simulink model "CircuitoGlobal"  (R2018a)
settings: Solver=VariableStepAuto  StartTime=0.0  StopTime=10.0  RelTol=1e-3
libraries: powerlib x4, pePwmGenerator x1, simulink_extras x1
settings Model: Creator=MATHEUS  LastModifiedBy=MATHEUS

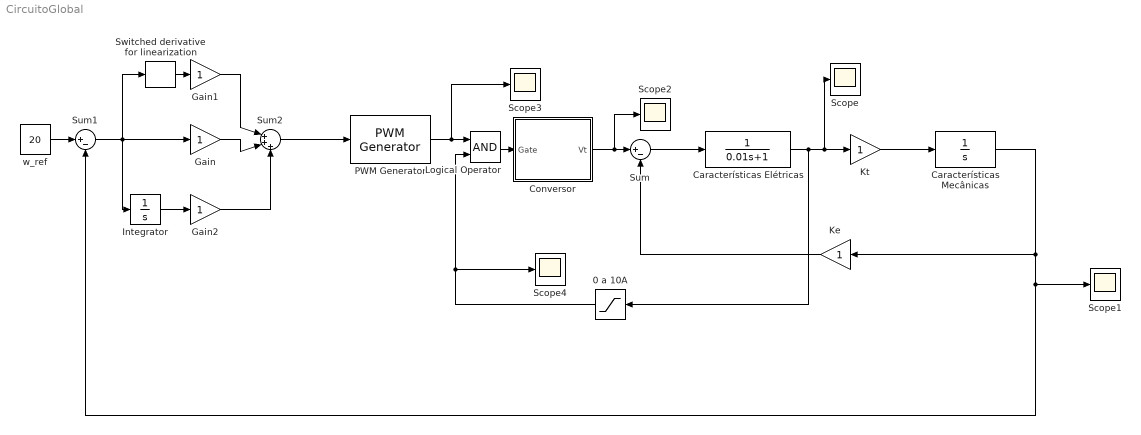
== system CircuitoGlobal ==
  0 a 10A : Saturate  UpperLimit=10  LowerLimit=0
  Características Elétricas : TransferFcn  Denominator=[0.01 1]
  "Características Mecânicas " : TransferFcn  Denominator=[1 0]
  Conversor : Subsystem
  Gain : Gain
  Gain1 : Gain
  Gain2 : Gain
  Integrator : Integrator
  Ke : Gain
  "Kt " : Gain
  Logical Operator : Logic  AllPortsSameDT=off  OutDataTypeStr=boolean
  PWM Generator : pePwmGenerator/PWM Generator  CarrCount=Up  Tper=2  Ts=0.01
  Scope{,1..4} (5 alike) : Scope
  Sum : Sum  Inputs=|+-
  Sum1 : Sum  Inputs=|+-
  Sum2 : Sum  Inputs=|+++
  Switched derivative for linearization : simulink_extras/Linearization/Switched derivative for linearization  switchVal=0  derivConst=100
      settings: SourceProductName=Simulink  SourceProductBaseCode=SL
  w_ref : Constant  Value=20
  wires:
  Conversor/1("Vt ") -> Scope2/1, Sum/1
  Sum/1 -> Características Elétricas/1
  Características Elétricas/1 -> 0 a 10A/1, Scope/1, "Kt "/1
  "Kt "/1 -> "Características Mecânicas "/1
  "Características Mecânicas "/1 -> Ke/1, Sum1/2, Scope1/1
  Ke/1 -> Sum/2
  Logical Operator/1 -> Conversor/1(Gate)
  Sum2/1 -> PWM Generator/1
  PWM Generator/1 -> Scope3/1, Logical Operator/1
  0 a 10A/1 -> Scope4/1, Logical Operator/2
  Sum1/1 -> Integrator/1, Switched derivative for linearization/1, Gain/1
  w_ref/1 -> Sum1/1
  Gain1/1 -> Sum2/1
  Gain/1 -> Sum2/2
  Gain2/1 -> Sum2/3
  Switched derivative for linearization/1 -> Gain1/1
  Integrator/1 -> Gain2/1

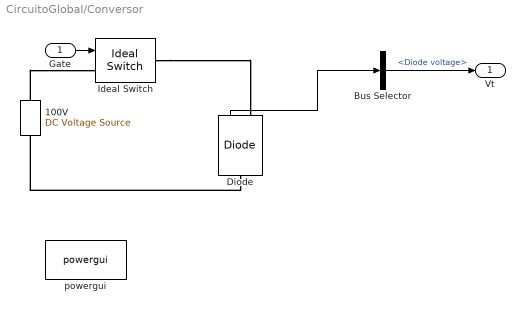
== system CircuitoGlobal/Conversor ==
  Gate : Inport
  100V : powerlib/Electrical Sources/DC Voltage Source  Amplitude=100  Measurements=None
      settings: SourceProductName=Simscape Electrical
  Bus Selector : BusSelector  OutputSignals=Diode voltage
  Diode : powerlib/Power Electronics/Diode  Ron=0.001  Lon=0  Vf=0.8  IC=0  UseSnubber=0  Rs=500  Cs=250e-9  Measurements=on
      settings: SourceProductName=Simscape Electrical
  Ideal Switch : powerlib/Power Electronics/Ideal Switch  Ron=0.001  Lon=0  IC=0  Rs=1e5  Cs=inf  Measurements=off
      settings: SourceProductName=Simscape Electrical
  powergui : powerlib/powergui  Priority=1  SimulationMode=Continuous  SampleTime=50e-6  frequency=60  Iterations=50  frequencyindice=0  Pbase=100e6  ErrMax=1e-4  UnitsV=kV  UnitsW=MW  buscounter=0  FunctionMessages=off  echomessages=off  EnableUseOfTLC=off  CurrentSourceSwitches=off  DisableSnubberDevices=off  DisableRonSwitches=off  DisableVfSwitches=off  DisplayEquations=off  SolverType=Tustin/Backward Euler (TBE)  Interpol=off  ExternalGateDelay=off  methode=off  Ts=100  x0status=blocks  SPID=on  SwTol=0  HookPort=off  RestoreLinks=warning  ResistiveCurrentMeasurement=off  Frange=[0:2:500]  Ylog=off  Xlog=on  ShowGrid=off  save=off  variable=ZData  structure=0  ZoomFFT=off  StartTime=0.0  cycles=1  DisplayStyle=1  fundamental=60  FreqAxis=off  MaxFrequency=1000  frequencyindicesteady=1  RmsSteady=1  display=off
      settings: SourceProductName=Simscape Electrical
  "Vt " : Outport
  wires:
  Gate/1 -> Ideal Switch/1
  Diode/1 -> Bus Selector/1
  Bus Selector/1 -> "Vt "/1  "<Diode voltage>"
  connections:
  Ideal Switch/RConn1 -- Diode/RConn1
  Diode/LConn1 -- 100V/LConn1
  100V/RConn1 -- Ideal Switch/LConn1
